simulink model "MidSpeedScada_Top"  (R2016b)
settings: Solver=VariableStepAuto  StartTime=0.0  StopTime=100.0  RelTol=1e-3
InitFcn:
  | InitialParam
values from neighbouring files (symbols this model uses):
  aRRC = 0.25    [InitialParam.m]
  BB_OSR = 8    [InitialParam.m]
  FsIF = FsBB * IF_OSR    (= 2880000)    [InitialParam.m]
  IF_OSR = 36    [InitialParam.m]
  nTSHead = 50    [InitialParam.m]
  Rs = 10e3    (= 10000)    [InitialParam.m]
  rxcFreq = 100e3    (= 100000)    [InitialParam.m]
  rxcPhi0 = pi/3    (= 1.0471975512)    [InitialParam.m]
  TFrame = 0.02    [InitialParam.m]
  txcFreq = txcFreq + (txcVCO / 1e6)*txcPPM    (= 100300)    [InitialParam.m]
  txcPhi0 = 0    [InitialParam.m]
libraries: dspsigops x4, commfilt2 x4, dsparch4 x4, commdigbbndam3 x3, dspsrcs4 x2, commrandsrc3 x1, commchan3 x1
settings Model: Creator=mizwong  LastModifiedBy=mizwong

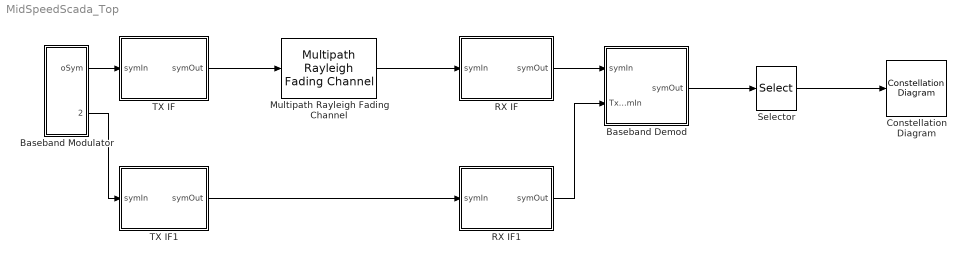
== system MidSpeedScada_Top ==
  Baseband Demod : Subsystem
  Baseband Modulator : Subsystem
  Constellation Diagram : ConstellationDiagram
  Multipath Rayleigh Fading Channel : commchan3/Multipath Rayleigh Fading Channel  maxDopplerShift=fd  spectrumType=Jakes  sigmaGaussian=1/sqrt(2)  coeffRounded=[1 -1.72 0.785]  freqMinMaxRJakes=[0 1]  freqMinMaxAJakes=[0 1]  sigmaGaussian1=1/sqrt(2)  sigmaGaussian2=1/sqrt(2)  centerFreqGaussian1=0.0  centerFreqGaussian2=0.0  gainGaussian1=0.5  gainGaussian2=0.5  coeffBell=9  dopplerSpectrum=doppler.jakes  pathDelays=tau  avgPathGaindB=pdb  normalizePathGains=on  seed=73  enableProbe=0  openVisAtStart=off  outPathGains=off  outDelay=off
  RX IF : Subsystem
  RX IF1 : Subsystem
  Selector : Selector  InputPortWidth=Rs*TFrame  IndexOptions=Index vector (dialog)  Indices=[nTSHead+1:Rs*TFrame]  OutputSizes=1
  TX IF : Subsystem
  TX IF1 : Subsystem
  wires:
  Baseband Modulator/1(oSym) -> TX IF/1(symIn)
  RX IF/1(symOut) -> Baseband Demod/1(symIn)
  TX IF1/1(symOut) -> RX IF1/1(symIn)
  Baseband Modulator/2(oTsSym) -> TX IF1/1(symIn)
  RX IF1/1(symOut) -> Baseband Demod/2(TxSymIn)
  Baseband Demod/1(symOut) -> Selector/1
  Selector/1 -> Constellation Diagram/1
  TX IF/1(symOut) -> Multipath Rayleigh Fading Channel/1
  Multipath Rayleigh Fading Channel/1 -> RX IF/1(symIn)

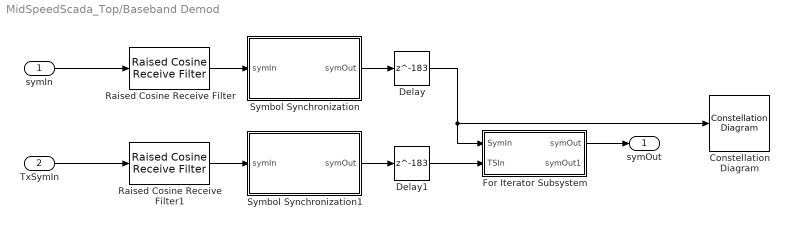
== system MidSpeedScada_Top/Baseband Demod ==
  symIn : Inport
  TxSymIn : Inport  Port=2
  Constellation Diagram : ConstellationDiagram
  Delay : Delay  DelayLength=183  InitialCondition=1  InputProcessing=Columns as channels (frame based)  SampleTime=1/Rs
  Delay1 : Delay  DelayLength=183  InitialCondition=1  InputProcessing=Columns as channels (frame based)  SampleTime=1/Rs
  For Iterator Subsystem : Subsystem  TreatAsAtomicUnit=on
  Raised Cosine Receive Filter : commfilt2/Raised Cosine Receive Filter  filtType=Square root  R=aRRC  filtSpan=16  N=BB_OSR  downFactor=1  downOffset=0  filterGain=1  InputProcessing=Columns as channels (frame based)  RateOptions=Allow multirate processing  framing=Mute  checkCoeff=off  variableName=rcRxFilt  currentFiltSpan=16  D=(16)/2  inputOffset=0  sampMode=Mute  saveAsFlag=0  rateMode=Downsampling  checkGain=Normalized  launchFVT=on  roundingMode=Floor  overflowMode=off  coeffDataTypeStr=Inherit: Same word length as input  coeffMin=[]  coeffMax=[]  coeffLastDataTypeStr=Inherit: Same word length as input  accumDataTypeStr=Inherit: Same as product output  accumLastDataTypeStr=Inherit: Same as product output  outputDataTypeStr=Inherit: Same as accumulator  outputMin=[]  outputMax=[]  outputLastDataTypeStr=Inherit: Same as accumulator
  Raised Cosine Receive Filter1 : commfilt2/Raised Cosine Receive Filter  filtType=Square root  R=aRRC  filtSpan=16  N=BB_OSR  downFactor=1  downOffset=0  filterGain=1  InputProcessing=Columns as channels (frame based)  RateOptions=Allow multirate processing  framing=Mute  checkCoeff=off  variableName=rcRxFilt1  currentFiltSpan=16  D=(16)/2  inputOffset=0  sampMode=Mute  saveAsFlag=0  rateMode=Downsampling  checkGain=Normalized  launchFVT=on  roundingMode=Floor  overflowMode=off  coeffDataTypeStr=Inherit: Same word length as input  coeffMin=[]  coeffMax=[]  coeffLastDataTypeStr=Inherit: Same word length as input  accumDataTypeStr=Inherit: Same as product output  accumLastDataTypeStr=Inherit: Same as product output  outputDataTypeStr=Inherit: Same as accumulator  outputMin=[]  outputMax=[]  outputLastDataTypeStr=Inherit: Same as accumulator
  Symbol Synchronization : Subsystem
  Symbol Synchronization1 : Subsystem
  symOut : Outport
  wires:
  symIn/1 -> Raised Cosine Receive Filter/1
  Raised Cosine Receive Filter/1 -> Symbol Synchronization/1(symIn)
  TxSymIn/1 -> Raised Cosine Receive Filter1/1
  Raised Cosine Receive Filter1/1 -> Symbol Synchronization1/1(symIn)
  For Iterator Subsystem/1(symOut) -> symOut/1
  Symbol Synchronization/1(symOut) -> Delay/1
  Symbol Synchronization1/1(symOut) -> Delay1/1
  Delay/1 -> For Iterator Subsystem/1(SymIn), Constellation Diagram/1
  Delay1/1 -> For Iterator Subsystem/2(TSIn)

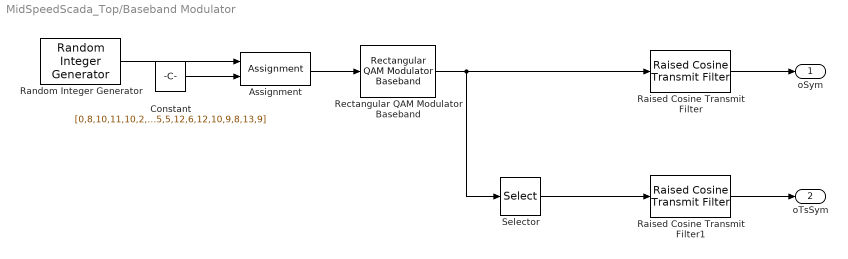
== system MidSpeedScada_Top/Baseband Modulator ==
  Assignment : Assignment  DiagnosticForDimensions=Warning  IndexOptions=Index vector (dialog)  Indices=[1:nTSHead]  OutputSizes=1
  Constant : Constant  Value=[0,8,10,11,10,2,12,5,8,5,4,2,4,7,9,0,5,0,11,6,9,1,10,7,11,2,5,4,14,4,0,1,5,6,7,11,7,5,1,1,5,5,12,6,12,10,9,8,13,9]
  Raised Cosine Transmit Filter : commfilt2/Raised Cosine Transmit Filter  filtType=Square root  R=aRRC  filtSpan=16  N=BB_OSR  filterGain=1  InputProcessing=Columns as channels (frame based)  RateOptions=Enforce single-rate processing  framing=Mute  checkCoeff=off  variableName=rcTxFilt  checkGain=Normalized  sampMode=Mute  saveAsFlag=0  currentFiltSpan=16  D=(16)/2  launchFVT=on  roundingMode=Floor  overflowMode=off  coeffDataTypeStr=Inherit: Same word length as input  coeffMin=[]  coeffMax=[]  coeffLastDataTypeStr=Inherit: Same word length as input  outputDataTypeStr=Inherit: Same as accumulator  outputMin=[]  outputMax=[]  outputLastDataTypeStr=Inherit: Same as accumulator
  Raised Cosine Transmit Filter1 : commfilt2/Raised Cosine Transmit Filter  filtType=Square root  R=aRRC  filtSpan=16  N=BB_OSR  filterGain=1  InputProcessing=Columns as channels (frame based)  RateOptions=Enforce single-rate processing  framing=Mute  checkCoeff=off  variableName=rcTxFilt1  checkGain=Normalized  sampMode=Mute  saveAsFlag=0  currentFiltSpan=16  D=(16)/2  launchFVT=on  roundingMode=Floor  overflowMode=off  coeffDataTypeStr=Inherit: Same word length as input  coeffMin=[]  coeffMax=[]  coeffLastDataTypeStr=Inherit: Same word length as input  outputDataTypeStr=Inherit: Same as accumulator  outputMin=[]  outputMax=[]  outputLastDataTypeStr=Inherit: Same as accumulator
  Random Integer Generator : commrandsrc3/Random Integer Generator  SetSize=M  SeedSource=Auto  Seed=0  SampleTime=1/Rs  SamplesPerFrame=TFrame*Rs  OutputDataType=double  SimulateUsing=Interpreted execution
  Rectangular QAM Modulator Baseband : commdigbbndam3/Rectangular QAM Modulator Baseband  M=M  InType=Integer  Enc=Gray  Mapping=[0:15]  PowType=Min. distance between symbols  MinDist=2  AvgPow=1  PeakPow=1  Ph=0  outDtype=double  outWordLen=16  outUDDataType=sfix(16)  outFracLenMode=Best precision  outFracLen=15  outDataTypeStr=double  outLastDataTypeStr=double
  Selector : Selector  InputPortWidth=TFrame*Rs  IndexOptions=Index vector (dialog)  Indices=[1:nTSHead]  OutputSizes=1
  oSym : Outport
  oTsSym : Outport  Port=2
  wires:
  Random Integer Generator/1 -> Assignment/1
  Raised Cosine Transmit Filter/1 -> oSym/1
  Raised Cosine Transmit Filter1/1 -> oTsSym/1
  Constant/1 -> Assignment/2
  Assignment/1 -> Rectangular QAM Modulator Baseband/1
  Selector/1 -> Raised Cosine Transmit Filter1/1
  Rectangular QAM Modulator Baseband/1 -> Raised Cosine Transmit Filter/1, Selector/1

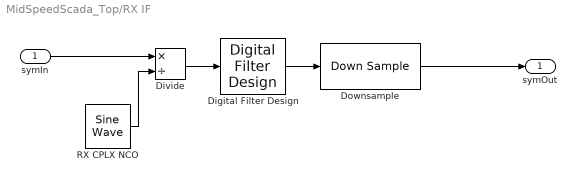
== system MidSpeedScada_Top/RX IF ==
  symIn : Inport
  Digital Filter Design : dsparch4/Digital Filter Design  mwdsp_browser_bugfix_var=off
  Divide : Product  Inputs=*/
  Downsample : DownSample  N=IF_OSR
  RX CPLX NCO : dspsrcs4/Sine Wave  Amplitude=1  Frequency=rxcFreq  Phase=2*pi*rxcPhi0  SampleMode=Discrete  OutComplex=Complex  CompMethod=Trigonometric fcn  TableSize=Speed  SampleTime=1/FsIF  SamplesPerFrame=TFrame*FsIF  ResetState=Restart at time zero  OutputFrames=off  dataType=double  wordLen=16  udDataType=sfix(16)  fracBitsMode=Best precision  numFracBits=15  OutDataTypeStr=double  LastOutDataTypeStr=double
  symOut : Outport
  wires:
  RX CPLX NCO/1 -> Divide/2
  Downsample/1 -> symOut/1
  Digital Filter Design/1 -> Downsample/1
  symIn/1 -> Divide/1
  Divide/1 -> Digital Filter Design/1

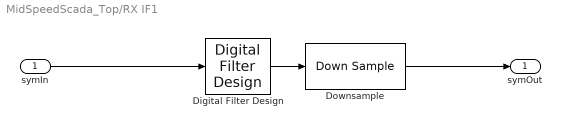
== system MidSpeedScada_Top/RX IF1 ==
  symIn : Inport
  Digital Filter Design : dsparch4/Digital Filter Design  mwdsp_browser_bugfix_var=off
  Downsample : DownSample  N=IF_OSR
  symOut : Outport
  wires:
  Downsample/1 -> symOut/1
  Digital Filter Design/1 -> Downsample/1
  symIn/1 -> Digital Filter Design/1

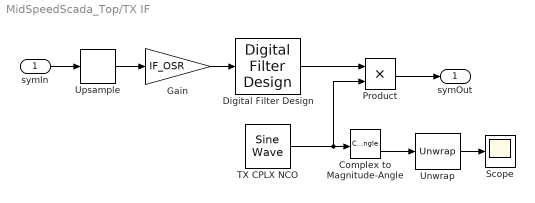
== system MidSpeedScada_Top/TX IF ==
  symIn : Inport
  Complex to Magnitude-Angle : ComplexToMagnitudeAngle
  Digital Filter Design : dsparch4/Digital Filter Design  mwdsp_browser_bugfix_var=off
  Gain : Gain  Gain=IF_OSR
  Product : Product
  Scope : Scope
  TX CPLX NCO : dspsrcs4/Sine Wave  Amplitude=1  Frequency=txcFreq  Phase=2*pi*txcPhi0  SampleMode=Discrete  OutComplex=Complex  CompMethod=Trigonometric fcn  TableSize=Speed  SampleTime=1/FsIF  SamplesPerFrame=TFrame*FsIF  ResetState=Restart at time zero  OutputFrames=off  dataType=double  wordLen=16  udDataType=sfix(16)  fracBitsMode=Best precision  numFracBits=15  OutDataTypeStr=double  LastOutDataTypeStr=double
  Unwrap : dspsigops/Unwrap  tol=pi  InputProcessing=Columns as channels (frame based)  running=off
  Upsample : dspsigops/Upsample  N=IF_OSR  phase=0  InputProcessing=Columns as channels (frame based)  RateOptions=Enforce single-rate processing  ic=0  mode=Unused parameter value
  symOut : Outport
  wires:
  Gain/1 -> Digital Filter Design/1
  TX CPLX NCO/1 -> Complex to Magnitude-Angle/1, Product/2
  Product/1 -> symOut/1
  Digital Filter Design/1 -> Product/1
  Upsample/1 -> Gain/1
  symIn/1 -> Upsample/1
  Unwrap/1 -> Scope/1
  Complex to Magnitude-Angle/2 -> Unwrap/1

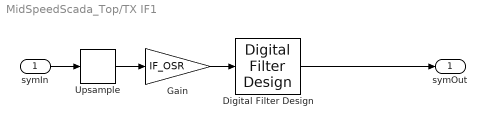
== system MidSpeedScada_Top/TX IF1 ==
  symIn : Inport
  Digital Filter Design : dsparch4/Digital Filter Design  mwdsp_browser_bugfix_var=off
  Gain : Gain  Gain=IF_OSR
  Upsample : dspsigops/Upsample  N=IF_OSR  phase=0  InputProcessing=Columns as channels (frame based)  RateOptions=Enforce single-rate processing  ic=0  mode=Unused parameter value
  symOut : Outport
  wires:
  Gain/1 -> Digital Filter Design/1
  Digital Filter Design/1 -> symOut/1
  Upsample/1 -> Gain/1
  symIn/1 -> Upsample/1

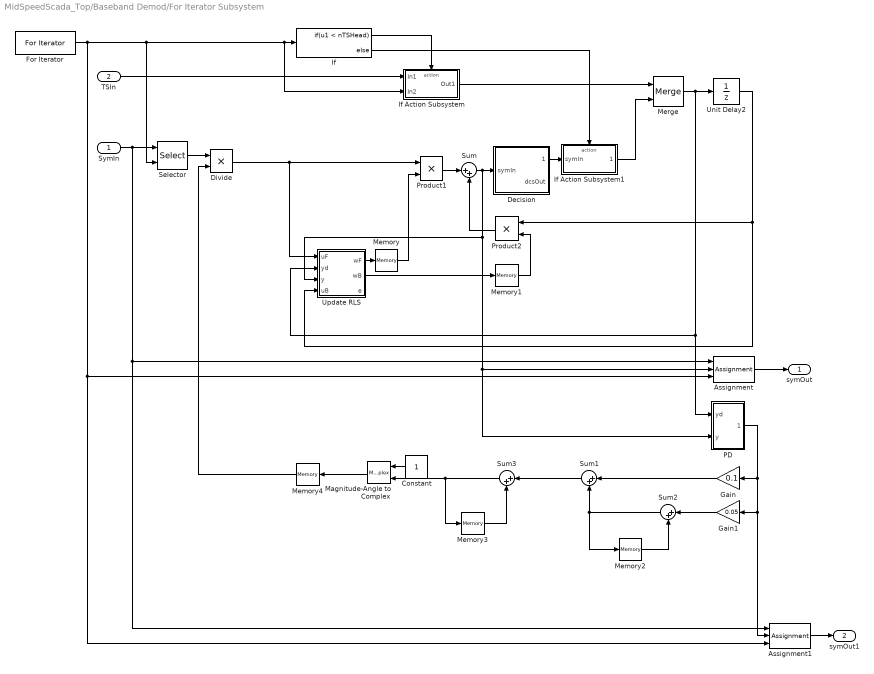
== system MidSpeedScada_Top/Baseband Demod/For Iterator Subsystem ==
  SymIn : Inport
  TSIn : Inport  Port=2
  Assignment : Assignment  DiagnosticForDimensions=Warning  IndexOptions=Index vector (port)  Indices=1  OutputSizes=1
  Assignment1 : Assignment  DiagnosticForDimensions=Warning  IndexOptions=Index vector (port)  Indices=1  OutputSizes=1
  Constant : Constant
  Decision : Subsystem
  Divide : Product  Inputs=**
  For Iterator : ForIterator  IterationLimit=Rs*TFrame
  Gain : Gain  Gain=0.1
  Gain1 : Gain  Gain=0.05
  If : If  IfExpression=u1 < nTSHead
  If Action Subsystem : Subsystem  TreatAsAtomicUnit=on
  If Action Subsystem1 : Subsystem  TreatAsAtomicUnit=on
  Magnitude-Angle to Complex : MagnitudeAngleToComplex
  Memory : Memory  X0=1  InheritSampleTime=on
  Memory1 : Memory  X0=1  InheritSampleTime=on
  Memory2 : Memory  InheritSampleTime=on
  Memory3 : Memory  InheritSampleTime=on
  Memory4 : Memory  X0=1  InheritSampleTime=on
  Merge : Merge
  PD : Subsystem
  Product1 : Product
  Product2 : Product
  Selector : Selector  InputPortWidth=Rs*TFrame  IndexOptions=Index vector (port)  Indices=[1 3]  OutputSizes=1
  Sum{,1..3} (4 alike) : Sum  Inputs=|++
  Unit Delay2 : UnitDelay  SampleTime=-1
  Update RLS : Stateflow chart  TreatAsAtomicUnit=on
  symOut : Outport
  symOut1 : Outport  Port=2
  wires:
  TSIn/1 -> If Action Subsystem/1(In1)
  If/1 -> If Action Subsystem/Action
  If Action Subsystem/1(Out1) -> Merge/1
  For Iterator/1 -> If Action Subsystem/2(In2), If/1, Selector/2, Assignment1/3, Assignment/3
  Divide/1 -> Update RLS/1(uF), Product1/1
  If Action Subsystem1/1(symOut) -> Merge/2
  If/2 -> If Action Subsystem1/Action
  Sum/1 -> Decision/1(symIn), PD/2(y), Assignment/2, Update RLS/3(y)
  Merge/1 -> Unit Delay2/1, PD/1(yd), Update RLS/2(yd)
  Assignment/1 -> symOut/1
  Update RLS/2(wB) -> Memory1/1
  Product1/1 -> Sum/1
  Update RLS/1(wF) -> Memory/1
  Product2/1 -> Sum/2
  Unit Delay2/1 -> Update RLS/4(uB), Product2/1
  Decision/1(symOut) -> If Action Subsystem1/1(symIn)
  PD/1(ePhi) -> Assignment1/2, Gain1/1, Gain/1
  Gain/1 -> Sum1/1
  Sum2/1 -> Sum1/2, Memory2/1
  Sum1/1 -> Sum3/1
  Sum3/1 -> Memory3/1, Magnitude-Angle to Complex/2
  Constant/1 -> Magnitude-Angle to Complex/1
  Selector/1 -> Divide/1
  Memory2/1 -> Sum2/2
  Memory3/1 -> Sum3/2
  Magnitude-Angle to Complex/1 -> Memory4/1
  Gain1/1 -> Sum2/1
  SymIn/1 -> Assignment1/1, Assignment/1, Selector/1
  Assignment1/1 -> symOut1/1
  Memory/1 -> Product1/2
  Memory4/1 -> Divide/2
  Memory1/1 -> Product2/2

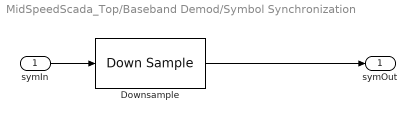
== system MidSpeedScada_Top/Baseband Demod/Symbol Synchronization ==
  symIn : Inport
  Downsample : DownSample  N=BB_OSR  phase=1
  symOut : Outport
  wires:
  symIn/1 -> Downsample/1
  Downsample/1 -> symOut/1

== system MidSpeedScada_Top/Baseband Demod/Symbol Synchronization1 ==
  symIn : Inport
  Downsample : DownSample  N=BB_OSR  phase=1
  symOut : Outport
  wires:
  symIn/1 -> Downsample/1
  Downsample/1 -> symOut/1

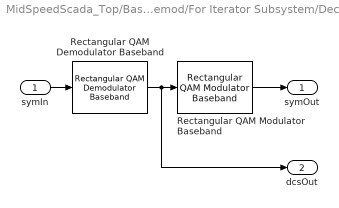
== system MidSpeedScada_Top/Baseband Demod/For Iterator Subsystem/Decision ==
  symIn : Inport
  Rectangular QAM Demodulator Baseband : commdigbbndam3/Rectangular QAM Demodulator Baseband  M=M  OutType=Bit  DecType=Hard decision  VarSource=Dialog  Variance=1  Dec=Gray  Mapping=[0:15]  PowType=Min. distance between symbols  MinDist=2  AvgPow=1  PeakPow=1  Ph=0  outDtype1=Inherit via internal rule  outDtype2=Inherit via internal rule  derotateFactorWordLen=16  derotateFactorDataTypeStr=Inherit: Same word length as input  derotateFactorLastDataTypeStr=Inherit: Same word length as input  denormFactorWordLen=16  denormFactorDataTypeStr=Inherit: Same word length as input  denormFactorLastDataTypeStr=Inherit: Same word length as input  prodOutWordLen=32  prodOutOverflowMode=Wrap  prodOutRoundingMode=Floor  prodOutOvFlMode=off  prodOutOvFlModeLastStrValue=off  sumWordLen=32
  Rectangular QAM Modulator Baseband : commdigbbndam3/Rectangular QAM Modulator Baseband  M=M  InType=Bit  Enc=Gray  Mapping=[0:15]  PowType=Min. distance between symbols  MinDist=2  AvgPow=1  PeakPow=1  Ph=0  outDtype=double  outWordLen=16  outUDDataType=sfix(16)  outFracLenMode=Best precision  outFracLen=15  outDataTypeStr=double  outLastDataTypeStr=double
  symOut : Outport
  dcsOut : Outport  Port=2
  wires:
  Rectangular QAM Demodulator Baseband/1 -> dcsOut/1, Rectangular QAM Modulator Baseband/1
  Rectangular QAM Modulator Baseband/1 -> symOut/1
  symIn/1 -> Rectangular QAM Demodulator Baseband/1

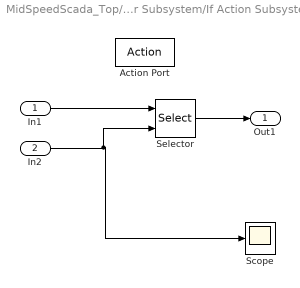
== system MidSpeedScada_Top/Baseband Demod/For Iterator Subsystem/If Action Subsystem ==
  In1 : Inport
  In2 : Inport  Port=2
  Action Port : ActionPort  ActionType=then
  Scope : Scope
  Selector : Selector  InputPortWidth=nTSHead  IndexOptions=Index vector (port)  Indices=[1 3]  OutputSizes=1
  Out1 : Outport
  wires:
  In1/1 -> Selector/1
  In2/1 -> Scope/1, Selector/2
  Selector/1 -> Out1/1

== system MidSpeedScada_Top/Baseband Demod/For Iterator Subsystem/If Action Subsystem1 ==
  symIn : Inport
  Action Port : ActionPort  ActionType=else
  symOut : Outport
  wires:
  symIn/1 -> symOut/1

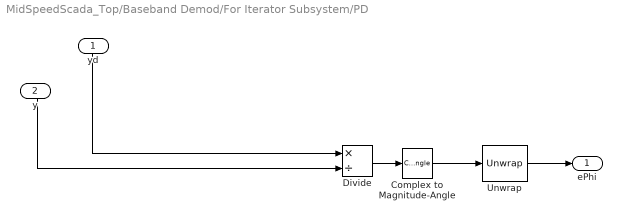
== system MidSpeedScada_Top/Baseband Demod/For Iterator Subsystem/PD ==
  yd : Inport
  y : Inport  Port=2
  Complex to Magnitude-Angle : ComplexToMagnitudeAngle  Output=Angle
  Divide : Product  Inputs=*/
  Unwrap : dspsigops/Unwrap  tol=pi  running=off
  ePhi : Outport
  wires:
  yd/1 -> Divide/1
  y/1 -> Divide/2
  Unwrap/1 -> ePhi/1
  Divide/1 -> Complex to Magnitude-Angle/1
  Complex to Magnitude-Angle/1 -> Unwrap/1

== stateflow chart MidSpeedScada_Top/Baseband Demod/For Iterator Subsystem/Update RLS ==
  state Initialize
    entry :
    P = (.1+0j)*eye(2);
    wF = 1+0j;
    wB = 1+0j;
    state = 1;
    w = [wF;wB];
    u=[uF;uB];
    K = P*u / (lamda+u'*P*u);
    P = (P-K*u'*P)/lamda;
    w = w + conj(K)*(yd-y);
    wF = w(1);
    wB = w(2);
  state Adapt
    entry:
    u=[uF;uB];
    K = P*u / (lamda+u'*P*u);
    P = (P-K*u'*P)/lamda;
    w = w + conj(K)*(yd-y);
    wF = w(1);
    wB = w(2);
    during:
    u=[uF;uB];
    K = P*u / (lamda+u'*P*u);
    P = (P-K*u'*P)/lamda;
    e = (yd-y);
    w = w + conj(K)*e;
    wF = w(1);
    wB = w(2);
  (default) -> Initialize
  Initialize -> Adapt : [state == 1]
  data: wF output; wB output; uF input; yd input; y input; P local; K local; lamda constant double =0.99; w local; state local =0; uB input; u local; e output
